simulink model "Simple_4Quad_payload_10_2017a"  (R2017a)
settings: Solver=ode45  StartTime=0.0  StopTime=100  FixedStep=0.001  RelTol=1e-3
InitFcn:
  | Simple_4Quad_payload_10_const
values from neighbouring files (symbols this model uses):
  All_rho = [d1 0 0 ... (first row only)    [Colab_4Quad_model_01_const.m]    (also in Colab_4Quad_model_02_const.m; Simple_4Quad_payload_04_const.m; Simple_4Quad_payload_05_const.m; Simple_4Quad_payload_06_const.m)
  alpha_chatt = 0.1    [Simple_4Quad_payload_09_const.m]    (also in Simple_4Quad_payload_10_const.m = 0.001; Simple_4Quad_payload_11_const.m = 0.01; Simple_4Quad_payload_12_const.m = 0.01)
  alphaTF = 0.1    [Simple_4Quad_payload_08_const.m]    (also in Simple_4Quad_payload_09_const.m = 0.5; Simple_4Quad_payload_10_const.m = 1; Simple_4Quad_payload_11_const.m = 0.5; Simple_4Quad_payload_12_const.m = 10)
  B_ob = [zeros(3);eye(3)]    [Simple_4Quad_payload_04_const.m]    (also in Simple_4Quad_payload_05_const.m; Simple_4Quad_payload_06_const.m; Simple_4Quad_payload_07_const.m; Simple_4Quad_payload_08_const.m)
  BBT_inv = ((B'*B)^(-1))*B'    [Simple_2Quad_payload_03_const.m]    (also in Simple_4Quad_payload_04_const.m = ((BR'*BR)^(-1))*BR'; Simple_4Quad_payload_05_const.m = ((BR'*BR)^(-1))*BR'; Simple_4Quad_payload_06_const.m = ((BR'*BR)^(-1))*BR'; Simple_4Quad_payload_07_const.m = ((BR'*BR)^(-1))*BR')
  BBT_invp = ((BRp'*BRp)^(-1))*BRp'    [Simple_4Quad_payload_10_const.m]    (also in Simple_4Quad_payload_11_const.m; Simple_4Quad_payload_12_const.m)
  BR = 1e0*eye(n)    [Simple_4Quad_payload_04_const.m]    (also in Simple_4Quad_payload_05_const.m; Simple_4Quad_payload_06_const.m; Simple_4Quad_payload_07_const.m; Simple_4Quad_payload_08_const.m)
  BRp = 1e0*eye(np)    [Simple_4Quad_payload_10_const.m]    (also in Simple_4Quad_payload_11_const.m; Simple_4Quad_payload_12_const.m)
  C_ob = [eye(3) zeros(3)]    [Simple_4Quad_payload_04_const.m]    (also in Simple_4Quad_payload_05_const.m; Simple_4Quad_payload_06_const.m; Simple_4Quad_payload_07_const.m; Simple_4Quad_payload_08_const.m)
  cons_sld = 0.001    [Simple_4Quad_payload_10_const.m]    (also in Simple_4Quad_payload_11_const.m = 0.01; Simple_4Quad_payload_12_const.m = 0.01)
  d1 = 0.25    [Colab_4Quad_model_01_const.m]    (also in Colab_4Quad_model_02_const.m = 0.5; Simple_4Quad_payload_01_const.m = 1; Simple_4Quad_payload_02_const.m = 1; Simple_4Quad_payload_03_const.m = 1)
  d2 = 0.25    [Colab_4Quad_model_01_const.m]    (also in Colab_4Quad_model_02_const.m = 0.5; Simple_4Quad_payload_01_const.m = 1; Simple_4Quad_payload_02_const.m = 1; Simple_4Quad_payload_03_const.m = 1)
  Des_rel_dist = 2    [Simple_4Quad_payload_01_const.m]    (also in Simple_4Quad_payload_02_const.m = 4; Simple_4Quad_payload_03_const.m = 4; Simple_4Quad_payload_04_const.m; Simple_4Quad_payload_05_const.m)
  g = 9.81    [Colab_4Quad_model_01_const.m]    (also in Colab_4Quad_model_02_const.m; Simple_2Quad_payload_01_const.m; Simple_2Quad_payload_02_const.m; Simple_2Quad_payload_03_const.m)
  gamma_0 = 1e-0*diag([1e-3;1e-0])    [Simple_2Quad_payload_03_const.m]    (also in Simple_4Quad_payload_04_const.m = 1e-0*diag([1e-6*ones(3,1);1e-0*ones(3,1)]); Simple_4Quad_payload_05_const.m = 1e-1*diag([1e-6*ones(3,1);1e-0*ones(3,1)]); Simple_4Quad_payload_06_const.m = 1e-0*diag([1e-6*ones(3,1);1e-0*ones(3,1)]); Simple_4Quad_payload_07_const.m = 1e-0*diag([1e-6*ones(3,1);1e-0*ones(3,1)]))
  gamma_0a = 1e-0*diag(1e-0*ones(3,1))    [Simple_4Quad_payload_10_const.m]    (also in Simple_4Quad_payload_11_const.m = 1e-0*diag(1e-6*ones(3,1)))
  gamma_0L = 1e-0*diag([1e-6*ones(3,1);1e-0*ones(3,1)])    [Simple_4Quad_payload_08_const.m]    (also in Simple_4Quad_payload_09_const.m; Simple_4Quad_payload_10_const.m = 1e+0*diag([1e-3*ones(3,1);1e-3*ones(3,1)]); Simple_4Quad_payload_11_const.m = 1e+0*diag([1e-3*ones(3,1);1e-3*ones(3,1)]); Simple_4Quad_payload_12_const.m = 1e+2*diag(1e-4*ones(3,1)))
  gamma_0p = 1e-0*diag(1e-3*ones(3,1))    [Simple_4Quad_payload_10_const.m]    (also in Simple_4Quad_payload_11_const.m = 1e-0*diag(1e-6*ones(3,1)))
  gamma_0r = 1e-0*diag(1e-3*ones(3,1))    [Simple_4Quad_payload_10_const.m]    (also in Simple_4Quad_payload_11_const.m = 1e-0*diag(1e-6*ones(3,1)); Simple_4Quad_payload_12_const.m = 1e+3*diag(1e-0*ones(3,1)))
  gamma_0v = 1e-0*diag([1e-0*ones(3,1);1e-0*ones(3,1)])    [Simple_4Quad_payload_08_const.m]    (also in Simple_4Quad_payload_09_const.m = 1e-0*diag([1e-6*ones(3,1);1e-6*ones(3,1)]); Simple_4Quad_payload_10_const.m = 1e+0*diag(1e-0*ones(3,1)); Simple_4Quad_payload_11_const.m = 1e+0*diag(1e-0*ones(3,1)); Simple_4Quad_payload_12_const.m = 1e+3*diag(1e-0*ones(3,1)))
  gamma_1 = 1e+2*diag([1e-3;1e-0])    [Simple_2Quad_payload_03_const.m]    (also in Simple_4Quad_payload_04_const.m = 1e+2*diag([1e-6*ones(3,1);1e-0*ones(3,1)]); Simple_4Quad_payload_05_const.m = 1e+2*diag([1e-6*ones(3,1);1e-0*ones(3,1)]); Simple_4Quad_payload_06_const.m = 1e+3*diag([1e-6*ones(3,1);1e-0*ones(3,1)]); Simple_4Quad_payload_07_const.m = 1e+3*diag([1e-6*ones(3,1);1e-0*ones(3,1)]))
  gamma_1a = 1e+0*diag(1e-0*ones(3,1))    [Simple_4Quad_payload_10_const.m]    (also in Simple_4Quad_payload_11_const.m = 1e+0*diag(1e-6*ones(3,1)))
  gamma_1L = 1e+3*diag([1e-6*ones(3,1);1e-0*ones(3,1)])    [Simple_4Quad_payload_08_const.m]    (also in Simple_4Quad_payload_09_const.m = 1e+2*diag([1e-6*ones(3,1);1e-0*ones(3,1)]); Simple_4Quad_payload_10_const.m = 1e+1*diag([1e-3*ones(3,1);1e-3*ones(3,1)]); Simple_4Quad_payload_11_const.m = 1e+0*diag([1e-3*ones(3,1);1e-3*ones(3,1)]); Simple_4Quad_payload_12_const.m = 1e+2*diag(1e-4*ones(3,1)))
  gamma_1p = 1e+0*diag(1e-3*ones(3,1))    [Simple_4Quad_payload_10_const.m]    (also in Simple_4Quad_payload_11_const.m = 1e+0*diag(1e-6*ones(3,1)))
  gamma_1r = 1e+0*diag(1e-3*ones(3,1))    [Simple_4Quad_payload_10_const.m]    (also in Simple_4Quad_payload_11_const.m = 1e+0*diag(1e-6*ones(3,1)); Simple_4Quad_payload_12_const.m = 1e+3*diag(1e-0*ones(3,1)))
  gamma_1v = 1e+3*diag([1e-0*ones(3,1);1e-0*ones(3,1)])    [Simple_4Quad_payload_08_const.m]    (also in Simple_4Quad_payload_09_const.m = 1e+2*diag([1e-6*ones(3,1);1e-6*ones(3,1)]); Simple_4Quad_payload_10_const.m = 1e+0*diag(1e-0*ones(3,1)); Simple_4Quad_payload_11_const.m = 1e+0*diag(1e-0*ones(3,1)); Simple_4Quad_payload_12_const.m = 1e+3*diag(1e-0*ones(3,1)))
  Ix = 0.166667    [Colab_4Quad_model_01_const.m]    (also in Colab_4Quad_model_02_const.m = 0.02; Simple_4Quad_payload_01_const.m = 1; Simple_4Quad_payload_02_const.m = 1; Simple_4Quad_payload_03_const.m = 1)
  Iy = 0.166667    [Colab_4Quad_model_01_const.m]    (also in Colab_4Quad_model_02_const.m = 0.02; Simple_4Quad_payload_01_const.m = 1; Simple_4Quad_payload_02_const.m = 1; Simple_4Quad_payload_03_const.m = 1)
  Iz = 0.166667    [Colab_4Quad_model_01_const.m]    (also in Colab_4Quad_model_02_const.m = 0.02; Simple_4Quad_payload_01_const.m = 1; Simple_4Quad_payload_02_const.m = 1; Simple_4Quad_payload_03_const.m = 1)
  Jo = diag([Ix;Iy;Iz])    [Colab_4Quad_model_01_const.m]    (also in Colab_4Quad_model_02_const.m; Simple_4Quad_payload_04_const.m; Simple_4Quad_payload_05_const.m; Simple_4Quad_payload_06_const.m)
  Jq = diag([0.0291 0.0291 0.0552])    [Colab_4Quad_model_01_const.m]    (also in Colab_4Quad_model_02_const.m = diag([0.03 0.03 0.06]); Simple_4Quad_payload_03_const.m = 1.2416e-3 * diag([1 1 2]); Simple_4Quad_payload_04_const.m = 1 * diag([1 1 2]); Simple_4Quad_payload_05_const.m = 1 * diag([1 1 2]))
  k1 = 1    [Simple_2Quad_payload_03_const.m]    (also in Simple_4Quad_payload_04_const.m; Simple_4Quad_payload_05_const.m; Simple_4Quad_payload_06_const.m; Simple_4Quad_payload_07_const.m)
  k2 = 0.1    [Simple_2Quad_payload_03_const.m]    (also in Simple_4Quad_payload_04_const.m; Simple_4Quad_payload_05_const.m; Simple_4Quad_payload_06_const.m; Simple_4Quad_payload_07_const.m)
  l = 3.1819    [Colab_4Quad_model_01_const.m]    (also in Colab_4Quad_model_02_const.m = 3; Simple_2Quad_payload_04_const.m = 1; Simple_4Quad_payload_01_const.m = 1; Simple_4Quad_payload_02_const.m = 2)
  m = 1.5    [Colab_4Quad_model_01_const.m]    (also in Colab_4Quad_model_02_const.m; Simple_2Quad_payload_04_const.m = 1; Simple_4Quad_payload_01_const.m = 1; Simple_4Quad_payload_02_const.m = 1)
  M = 1.0    (= 1)    [Colab_4Quad_model_01_const.m]    (also in Colab_4Quad_model_02_const.m; Simple_2Quad_payload_01_const.m; Simple_2Quad_payload_02_const.m; Simple_2Quad_payload_03_const.m)
  n = 2    [Simple_2Quad_payload_03_const.m]    (also in Simple_4Quad_payload_03_const.m = 6; Simple_4Quad_payload_04_const.m = 6; Simple_4Quad_payload_05_const.m = 6; Simple_4Quad_payload_06_const.m = 6)
  noise_var_RelAcc = 0e-6    (= 0)    [Simple_4Quad_payload_07_const.m]    (also in Simple_4Quad_payload_08_const.m; Simple_4Quad_payload_09_const.m; Simple_4Quad_payload_10_const.m; Simple_4Quad_payload_11_const.m)
  noise_var_RelPos = 0e-6    (= 0)    [Simple_4Quad_payload_07_const.m]    (also in Simple_4Quad_payload_08_const.m; Simple_4Quad_payload_09_const.m; Simple_4Quad_payload_10_const.m; Simple_4Quad_payload_11_const.m)
  np = 3    [Simple_4Quad_payload_10_const.m]    (also in Simple_4Quad_payload_11_const.m; Simple_4Quad_payload_12_const.m; constant_CAMFC2_Quad_New_02_Payload_01.m = 6)
  Q_ob = var_u_ob * eye(6)    [Simple_4Quad_payload_04_const.m]    (also in Simple_4Quad_payload_05_const.m; Simple_4Quad_payload_06_const.m; Simple_4Quad_payload_07_const.m; Simple_4Quad_payload_08_const.m)
  Qa = 1e-0*eye(np)    [Simple_4Quad_payload_10_const.m]    (also in Simple_4Quad_payload_11_const.m)
  QL = 1e-0*eye(n)    [Simple_4Quad_payload_08_const.m]    (also in Simple_4Quad_payload_09_const.m; Simple_4Quad_payload_10_const.m; Simple_4Quad_payload_11_const.m = 1e-2*eye(n); Simple_4Quad_payload_12_const.m = 1e-0*eye(np))
  Qp = 1e-0*eye(np)    [Simple_4Quad_payload_10_const.m]    (also in Simple_4Quad_payload_11_const.m = 1e-2*eye(np))
  QR = 1e-0*eye(n)    [Simple_4Quad_payload_04_const.m]    (also in Simple_4Quad_payload_05_const.m = 1e-1*eye(n); Simple_4Quad_payload_06_const.m; Simple_4Quad_payload_07_const.m; Simple_4Quad_payload_08_const.m)
  Qr = 1e-0*eye(np)    [Simple_4Quad_payload_10_const.m]    (also in Simple_4Quad_payload_11_const.m; Simple_4Quad_payload_12_const.m)
  Qv = 1e-0*eye(n)    [Simple_4Quad_payload_08_const.m]    (also in Simple_4Quad_payload_09_const.m; Simple_4Quad_payload_10_const.m = 1e-0*eye(np); Simple_4Quad_payload_11_const.m = 1e-2*eye(np); Simple_4Quad_payload_12_const.m = 1e-0*eye(np))
  R = 1e+0*eye(n)    [Simple_2Quad_payload_03_const.m]    (also in Simple_4Quad_payload_04_const.m = 1e+0*eye(m); Simple_4Quad_payload_05_const.m = 1e+0*eye(m); Simple_4Quad_payload_06_const.m; Simple_4Quad_payload_07_const.m)
  R_ob = var_y_ob * eye(3)    [Simple_4Quad_payload_04_const.m]    (also in Simple_4Quad_payload_05_const.m; Simple_4Quad_payload_06_const.m; Simple_4Quad_payload_07_const.m; Simple_4Quad_payload_08_const.m)
  rho_0 = 1e-0    (= 1)    [Simple_2Quad_payload_03_const.m]    (also in Simple_4Quad_payload_04_const.m; Simple_4Quad_payload_05_const.m = 0.1; Simple_4Quad_payload_06_const.m; Simple_4Quad_payload_07_const.m)
  rho_0a = 1e-0    (= 1)    [Simple_4Quad_payload_10_const.m]    (also in Simple_4Quad_payload_11_const.m)
  rho_0L = 1e-0    (= 1)    [Simple_4Quad_payload_08_const.m]    (also in Simple_4Quad_payload_09_const.m; Simple_4Quad_payload_10_const.m; Simple_4Quad_payload_11_const.m; Simple_4Quad_payload_12_const.m)
  rho_0p = 1e-0    (= 1)    [Simple_4Quad_payload_10_const.m]    (also in Simple_4Quad_payload_11_const.m)
  rho_0r = 1e-0    (= 1)    [Simple_4Quad_payload_10_const.m]    (also in Simple_4Quad_payload_11_const.m; Simple_4Quad_payload_12_const.m = 0.001)
  rho_0v = 1e-1    (= 0.1)    [Simple_4Quad_payload_08_const.m]    (also in Simple_4Quad_payload_09_const.m = 1; Simple_4Quad_payload_10_const.m = 1; Simple_4Quad_payload_11_const.m = 1; Simple_4Quad_payload_12_const.m = 1)
  rho_1 = 1e-0    (= 1)    [Simple_2Quad_payload_03_const.m]    (also in Simple_4Quad_payload_04_const.m; Simple_4Quad_payload_05_const.m; Simple_4Quad_payload_06_const.m; Simple_4Quad_payload_07_const.m)
  rho_1a = 1e-0    (= 1)    [Simple_4Quad_payload_10_const.m]    (also in Simple_4Quad_payload_11_const.m)
  rho_1L = 1e-0    (= 1)    [Simple_4Quad_payload_08_const.m]    (also in Simple_4Quad_payload_09_const.m; Simple_4Quad_payload_10_const.m; Simple_4Quad_payload_11_const.m; Simple_4Quad_payload_12_const.m)
  rho_1p = 1e-0    (= 1)    [Simple_4Quad_payload_10_const.m]    (also in Simple_4Quad_payload_11_const.m)
  rho_1r = 1e-0    (= 1)    [Simple_4Quad_payload_10_const.m]    (also in Simple_4Quad_payload_11_const.m; Simple_4Quad_payload_12_const.m)
  rho_1v = 1e-0    (= 1)    [Simple_4Quad_payload_08_const.m]    (also in Simple_4Quad_payload_09_const.m; Simple_4Quad_payload_10_const.m; Simple_4Quad_payload_11_const.m; Simple_4Quad_payload_12_const.m)
  Rp = 1e+0*eye(np)    [Simple_4Quad_payload_10_const.m]    (also in Simple_4Quad_payload_11_const.m; Simple_4Quad_payload_12_const.m)
  xo_init = 0    [Simple_4Quad_payload_10_const.m]    (also in Simple_4Quad_payload_11_const.m; Simple_4Quad_payload_12_const.m)
  yo_init = 0    [Simple_4Quad_payload_10_const.m]    (also in Simple_4Quad_payload_11_const.m; Simple_4Quad_payload_12_const.m)
  zo_init = 0    [Simple_4Quad_payload_10_const.m]    (also in Simple_4Quad_payload_11_const.m; Simple_4Quad_payload_12_const.m)
libraries: simulink x2
(part 5 of 5)

== matlab function Simple_4Quad_payload_10_2017a/Controllers and Observers/Controller - Payload/Payload_vel/g-Estimator1 ==
  data: sigma input; x input; P input; rho_0v parameter; gamma_0v parameter; Da_hat output; a_hat input
function Da_hat = fcn(sigma,x,P,rho_0v,gamma_0v,a_hat)

DVa_hat = - gamma_0v * P * diag(sigma) * (x - sigma) - rho_0v * gamma_0v * diag(a_hat);

Da_hat = diag(DVa_hat);

end

== matlab function Simple_4Quad_payload_10_2017a/Controllers and Observers/Controller - Payload/Payload_vel/main ==
  data: sigma input; zeta input; u output; Dy_d input; Rp parameter; P input; a_hat input; BRp parameter; g_hat input; x input; Qv parameter; BBT_invp parameter; np parameter
function u = fcn(sigma,zeta,Dy_d,Rp,P,a_hat,BRp,g_hat,x,Qv,BBT_invp,np)

u1 = (1/2) * Rp * BRp' * P * sigma;
u2 = BBT_invp * (Dy_d - a_hat*x + (eye(np) + 2*(((P)^(-1)*Qv)) + a_hat)*sigma - g_hat - zeta) - (3/4) * Rp * BRp' * P * sigma;

u = u1 + u2;

end

== matlab function Simple_4Quad_payload_10_2017a/Controllers and Observers/Controller - Payload/Payload_vel/variable change ==
  data: X input; Xd input; x_mod output; xd_mod output; e_mod output
function [x_mod,xd_mod,e_mod] = fcn(X,Xd)

x_mod = X;

xd_mod = Xd;

e_mod = xd_mod - x_mod;


end

== matlab function Simple_4Quad_payload_10_2017a/Controllers and Observers/Controller - Payload/Rotation_Q1/D Phi ==
  data: Omega_O input; D_PHI_O output; PHI_O input
function D_PHI_O = fcn(Omega_O,PHI_O)

phi_O = PHI_O(1);
theta_O = PHI_O(2);

Rm_O = [1 0 -sin(theta_O);
    0 cos(phi_O) cos(theta_O)*sin(phi_O);
    0 -sin(phi_O) cos(theta_O)*cos(phi_O)];

D_PHI_O = (Rm_O)^(-1) * Omega_O;


end

== matlab function Simple_4Quad_payload_10_2017a/Controllers and Observers/Controller - Payload/desired yaw ==
  data: P_des input; yaw_des output
function yaw_des = fcn(P_des)

yaw_des = atan2(P_des(1),-P_des(2));

end

== matlab function Simple_4Quad_payload_10_2017a/Controllers and Observers/Controller - Payload/Payload_att/CARE ==
  data: P input; a_hat input; BRp parameter; Rp parameter; DP output; Qa parameter
function DP = fcn(P,a_hat,BRp,Rp,Qa)

DP = a_hat*P + P*a_hat' - P*BRp*Rp*BRp'*P + 2*Qa;

end

== matlab function Simple_4Quad_payload_10_2017a/Controllers and Observers/Controller - Payload/Payload_att/Differentiator/Sliding differentiator ==
  data: u output; u1 input; e input; np parameter; k1 parameter; alpha_chatt parameter
function u = fcn(u1,e,np,k1,alpha_chatt)

b=k1;

ABS = zeros(np,1);
for i=1:np
    if e(i)>0
        ABS(i) = e(i);
    else
        ABS(i) = -e(i);
    end
end
SGN = e ./ (ABS + alpha_chatt);

u = u1 - b*(ABS.^0.5).*SGN;

end

== matlab function Simple_4Quad_payload_10_2017a/Controllers and Observers/Controller - Payload/Payload_att/Differentiator/Sliding differentiator1 ==
  data: Du1 output; e input; np parameter; k2 parameter; alpha_chatt parameter
function Du1 = fcn(e,np,k2,alpha_chatt)

a=k2;

ABS = zeros(np,1);
for i=1:np
    if e(i)>0
        ABS(i) = e(i);
    else
        ABS(i) = -e(i);
    end
end
SGN = e ./ (ABS + alpha_chatt);

Du1 = - a*SGN;

end

== matlab function Simple_4Quad_payload_10_2017a/Controllers and Observers/Controller - Payload/Payload_att/g-Estimator ==
  data: sigma input; g_hat input; P input; rho_1a parameter; gamma_1a parameter; Dg_hat output
function Dg_hat = fcn(sigma,g_hat,P,rho_1a,gamma_1a)

Dg_hat = - gamma_1a * P * sigma - rho_1a * gamma_1a * g_hat;

end

== matlab function Simple_4Quad_payload_10_2017a/Controllers and Observers/Controller - Payload/Payload_att/g-Estimator1 ==
  data: sigma input; x input; P input; rho_0a parameter; gamma_0a parameter; Da_hat output; a_hat input
function Da_hat = fcn(sigma,x,P,rho_0a,gamma_0a,a_hat)

DVa_hat = - gamma_0a * P * diag(sigma) * (x - sigma) - rho_0a * gamma_0a * diag(a_hat);

Da_hat = diag(DVa_hat);

end

== matlab function Simple_4Quad_payload_10_2017a/Controllers and Observers/Controller - Payload/Payload_att/main ==
  data: sigma input; zeta input; u output; Dy_d input; Rp parameter; P input; a_hat input; BRp parameter; g_hat input; x input; Qa parameter; BBT_invp parameter; np parameter
function u = fcn(sigma,zeta,Dy_d,Rp,P,a_hat,BRp,g_hat,x,Qa,BBT_invp,np)

u1 = (1/2) * Rp * BRp' * P * sigma;
u2 = BBT_invp * (Dy_d - a_hat*x + (eye(np) + 2*(((P)^(-1)*Qa)) + a_hat)*sigma - g_hat - zeta) - (3/4) * Rp * BRp' * P * sigma;

u = u1 + u2;

end

== matlab function Simple_4Quad_payload_10_2017a/Controllers and Observers/Controller - Payload/Payload_att/variable change ==
  data: X input; Xd input; x_mod output; xd_mod output; e_mod output
function [x_mod,xd_mod,e_mod] = fcn(X,Xd)

x_mod = X;

xd_mod = Xd;

e_mod = xd_mod - x_mod;


end

== matlab function Simple_4Quad_payload_10_2017a/Controllers and Observers/Controller - Payload/Payload_rate/CARE ==
  data: P input; a_hat input; BRp parameter; Rp parameter; DP output; Qr parameter
function DP = fcn(P,a_hat,BRp,Rp,Qr)

DP = a_hat*P + P*a_hat' - P*BRp*Rp*BRp'*P + 2*Qr;

end

== matlab function Simple_4Quad_payload_10_2017a/Controllers and Observers/Controller - Payload/Payload_rate/Differentiator/Sliding differentiator ==
  data: u output; u1 input; e input; np parameter; k1 parameter; alpha_chatt parameter
function u = fcn(u1,e,np,k1,alpha_chatt)

b=k1;

ABS = zeros(np,1);
for i=1:np
    if e(i)>0
        ABS(i) = e(i);
    else
        ABS(i) = -e(i);
    end
end
SGN = e ./ (ABS + alpha_chatt);

u = u1 - b*(ABS.^0.5).*SGN;

end

== matlab function Simple_4Quad_payload_10_2017a/Controllers and Observers/Controller - Payload/Payload_rate/Differentiator/Sliding differentiator1 ==
  data: Du1 output; e input; np parameter; k2 parameter; alpha_chatt parameter
function Du1 = fcn(e,np,k2,alpha_chatt)

a=k2;

ABS = zeros(np,1);
for i=1:np
    if e(i)>0
        ABS(i) = e(i);
    else
        ABS(i) = -e(i);
    end
end
SGN = e ./ (ABS + alpha_chatt);

Du1 = - a*SGN;

end

== matlab function Simple_4Quad_payload_10_2017a/Controllers and Observers/Controller - Payload/Payload_rate/g-Estimator ==
  data: sigma input; g_hat input; P input; rho_1r parameter; gamma_1r parameter; Dg_hat output
function Dg_hat = fcn(sigma,g_hat,P,rho_1r,gamma_1r)

Dg_hat = - gamma_1r * P * sigma - rho_1r * gamma_1r * g_hat;

end

== matlab function Simple_4Quad_payload_10_2017a/Controllers and Observers/Controller - Payload/Payload_rate/g-Estimator1 ==
  data: sigma input; x input; P input; rho_0r parameter; gamma_0r parameter; Da_hat output; a_hat input
function Da_hat = fcn(sigma,x,P,rho_0r,gamma_0r,a_hat)

DVa_hat = - gamma_0r * P * diag(sigma) * (x - sigma) - rho_0r * gamma_0r * diag(a_hat);

Da_hat = diag(DVa_hat);

end

== matlab function Simple_4Quad_payload_10_2017a/Controllers and Observers/Controller - Payload/Payload_rate/main ==
  data: sigma input; zeta input; u output; Dy_d input; Rp parameter; P input; a_hat input; BRp parameter; g_hat input; x input; Qr parameter; BBT_invp parameter; np parameter
function u = fcn(sigma,zeta,Dy_d,Rp,P,a_hat,BRp,g_hat,x,Qr,BBT_invp,np)

u1 = (1/2) * Rp * BRp' * P * sigma;
u2 = BBT_invp * (Dy_d - a_hat*x + (eye(np) + 2*(((P)^(-1)*Qr)) + a_hat)*sigma - g_hat - zeta) - (3/4) * Rp * BRp' * P * sigma;

u = u1 + u2;

end

== matlab function Simple_4Quad_payload_10_2017a/Controllers and Observers/Controller - Payload/Payload_rate/variable change ==
  data: X input; Xd input; x_mod output; xd_mod output; e_mod output
function [x_mod,xd_mod,e_mod] = fcn(X,Xd)

x_mod = X;

xd_mod = Xd;

e_mod = xd_mod - x_mod;


end
